simulink model "OswaldEProj1Sim"  (R2023a)
settings: Solver=VariableStepAuto  StartTime=0.0  StopTime=20  RelTol=1e-3
values from neighbouring files (symbols this model uses):
  DEG2RAD = pi/180    (= 0.0174532925199)    [OswaldEProj1Code.m]
  K_ari = -der.N_delta_a/der.N_delta_r    [OswaldEProj1Code.m]
  RAD2DEG = 180/pi    (= 57.2957795131)    [OswaldEProj1Code.m]
libraries: cstblocks x7
settings Model: Creator=ethan  LastModifiedBy=ethan

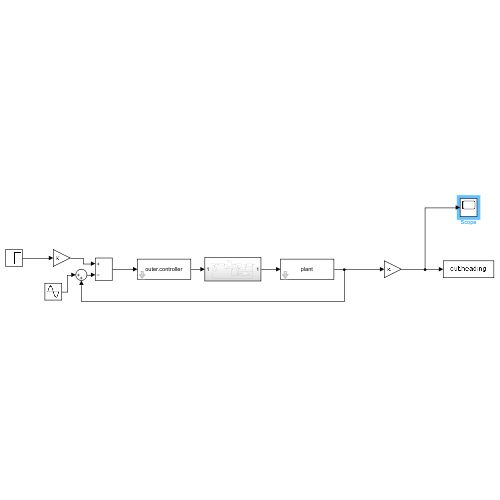
[thumbnail: Simulink's stored preview of the top-level diagram]
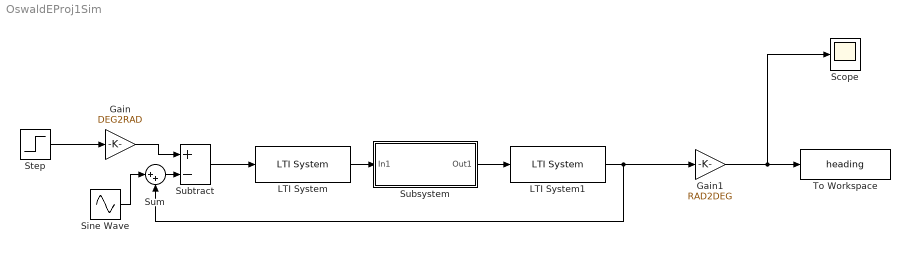
== system OswaldEProj1Sim ==
  Gain : Gain  Gain=DEG2RAD
  Gain1 : Gain  Gain=RAD2DEG
  LTI System : cstblocks/LTI System  sys=outer.controller  IC=[]
  LTI System1 : cstblocks/LTI System  sys=plant  IC=[]
  Scope : Scope
  Sine Wave : Sin  Amplitude=0.02  Frequency=100  SampleTime=0
  Step : Step  Time=0  After=5  SampleTime=0
  Subsystem : Subsystem
  Subtract : Sum  Inputs=+-
  Sum : Sum  Inputs=|++
  To Workspace : ToWorkspace  VariableName=heading  SaveFormat=Timeseries  SampleTime=-1
  wires:
  Step/1 -> Gain/1
  Subtract/1 -> LTI System/1
  LTI System/1 -> Subsystem/1(In1)
  Subsystem/1(Out1) -> LTI System1/1
  LTI System1/1 -> Gain1/1, Sum/2
  Sum/1 -> Subtract/2
  Sine Wave/1 -> Sum/1
  Gain/1 -> Subtract/1
  Gain1/1 -> Scope/1, To Workspace/1

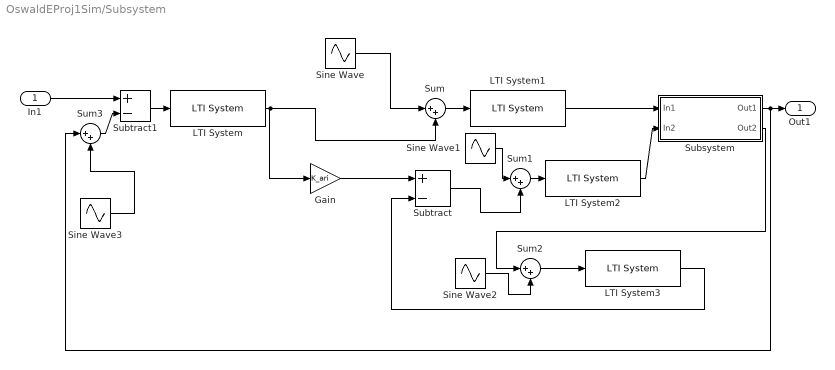
== system OswaldEProj1Sim/Subsystem ==
  In1 : Inport
  Gain : Gain  Gain=K_ari
  LTI System : cstblocks/LTI System  sys=inner.controller  IC=[]
  LTI System1 : cstblocks/LTI System  sys=actuator  IC=[]
  LTI System2 : cstblocks/LTI System  sys=actuator  IC=[]
  LTI System3 : cstblocks/LTI System  sys=K_r  IC=[]
  Sine Wave : Sin  Amplitude=0.01  SampleTime=0
  Sine Wave1 : Sin  Amplitude=0.01  SampleTime=0
  Sine Wave2 : Sin  Amplitude=0.05  Frequency=100  SampleTime=0
  Sine Wave3 : Sin  Amplitude=.02  Frequency=100  SampleTime=0
  Subsystem : Subsystem
  Subtract : Sum  Inputs=+-
  Subtract1 : Sum  Inputs=+-
  Sum{,1..3} (4 alike) : Sum  Inputs=|++
  Out1 : Outport
  wires:
  In1/1 -> Subtract1/1
  LTI System/1 -> Sum/2, Gain/1
  Gain/1 -> Subtract/1
  Subtract/1 -> Sum1/2
  Subsystem/1(Out1) -> Sum3/1, Out1/1
  Subsystem/2(Out2) -> Sum2/1
  Subtract1/1 -> LTI System/1
  Sine Wave/1 -> Sum/1
  Sine Wave1/1 -> Sum1/1
  Sum1/1 -> LTI System2/1
  Sine Wave2/1 -> Sum2/2
  Sum3/1 -> Subtract1/2
  Sine Wave3/1 -> Sum3/2
  LTI System1/1 -> Subsystem/1(In1)
  Sum/1 -> LTI System1/1
  LTI System2/1 -> Subsystem/2(In2)
  Sum2/1 -> LTI System3/1
  LTI System3/1 -> Subtract/2

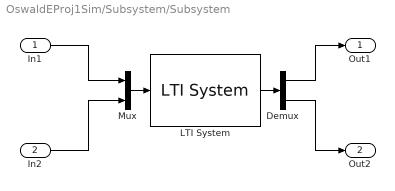
== system OswaldEProj1Sim/Subsystem/Subsystem ==
  In1 : Inport
  In2 : Inport  Port=2
  Demux : Demux  Outputs=2
  LTI System : cstblocks/LTI System  sys=G  IC=[]
  Mux : Mux  Inputs=2
  Out1 : Outport
  Out2 : Outport  Port=2
  wires:
  Demux/1 -> Out1/1
  Demux/2 -> Out2/1
  In2/1 -> Mux/2
  Mux/1 -> LTI System/1
  In1/1 -> Mux/1
  LTI System/1 -> Demux/1
